simulink model "Proportional_Control"  (R2022b)
settings: Solver=VariableStepAuto  StartTime=0.0  StopTime=10.0  RelTol=1e-3
settings Model: Creator=bekir  LastModifiedBy=bekir

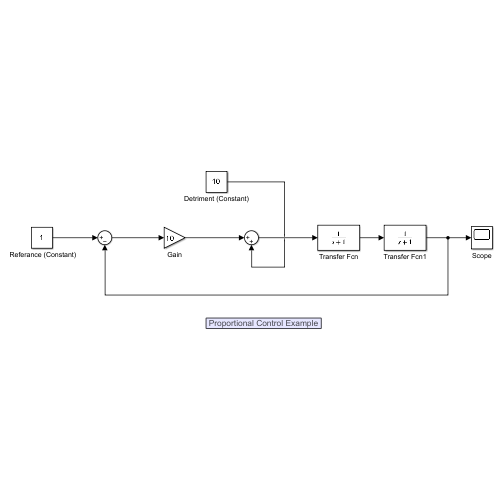
[thumbnail: Simulink's stored preview of the top-level diagram]
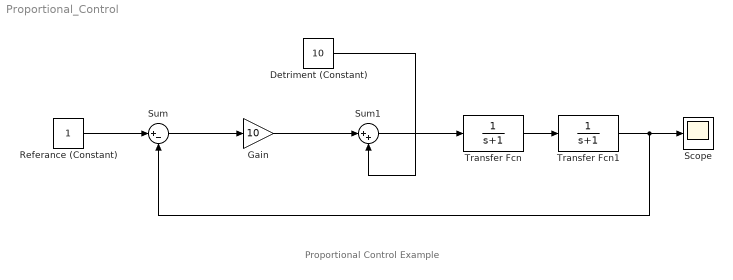
== system Proportional_Control ==
  note: Proportional Control Example
  " Referance (Constant)" : Constant
  Detriment (Constant) : Constant  Value=10
  Gain : Gain  Gain=10
  Scope : Scope
  Sum : Sum  Inputs=|+-
  Sum1 : Sum  Inputs=|++
  Transfer Fcn : TransferFcn  Denominator=[1 1]
  Transfer Fcn1 : TransferFcn  Denominator=[1 1]
  wires:
  Sum/1 -> Gain/1
  Sum1/1 -> Transfer Fcn/1
  Transfer Fcn/1 -> Transfer Fcn1/1
  Gain/1 -> Sum1/1
  Detriment (Constant)/1 -> Sum1/2
  Transfer Fcn1/1 -> Sum/2, Scope/1
  " Referance (Constant)"/1 -> Sum/1
